simulink model "Balancing_Logic"  (R2023b)
settings: Solver=FixedStepDiscrete  StartTime=0.0  StopTime=Inf  RelTol=1e-3  EnableMultiTasking=on
values from neighbouring files (symbols this model uses):
  BalNotActWait = 30    [DD_Balancing_Logic.sldd]
  BalOffWait = 20    [DD_Balancing_Logic.sldd]
  BalOnWait = 60    [DD_Balancing_Logic.sldd]
  flgEnBalancing = 1    [DD_Balancing_Logic.sldd]
  TargetDeltaV = 0.01    [DD_Balancing_Logic.sldd]
undefined symbols (not defined in the file or in its folder): Ns
settings Model: DataDictionary=DD_Balancing_Logic.sldd  ExtModeTrigDuration=8  Creator=cpatel  LastModifiedBy=Alkhouly
settings SolverCC: AlgebraicLoopSolver=TrustRegion  AutoInsertRateTranBlk=on
settings DataIOCC: ExternalInput=Battery  SaveOutput=off  SaveTime=off  SignalLoggingName=logsOut
settings OptimizationCC: UseDivisionForNetSlopeComputation=on  UseFloatMulNetSlope=on  DefaultUnderspecifiedDataType=single  UseSpecifiedMinMax=on  PassReuseOutputArgsAs=Individual arguments  NoFixptDivByZeroProtection=on  EfficientFloat2IntCast=on  LifeSpan=inf  MaxStackSize=1024  OptimizeBlockOrder=speed  DifferentSizesBufferReuse=on  EfficientTunableParamExpr=on
settings DebuggingCC: SignalInfNanChecking=error  SaveWithParameterizedLinksMsg=none  CheckExecutionContextPreStartOutputMsg=on  IntegerOverflowMsg=error  ParameterPrecisionLossMsg=none  ParameterTunabilityLossMsg=error  UnconnectedInputMsg=warning  UnconnectedOutputMsg=warning  UnconnectedLineMsg=warning  AssertControl=DisableAll  PregeneratedLibrarySubsystemCodeDiagnostic=none  SFUnexpectedBacktrackingDiag=warning  SFNoUnconditionalDefaultTransitionDiag=warning  SFExecutionAtInitializationDiag=none  ArithmeticOperatorsInVariantConditions=warning
settings HardwareCC: ProdBitPerChar=16  ProdBitPerInt=16  ProdBitPerPointer=32  ProdBitPerSizeT=32  ProdBitPerPtrDiffT=32  ProdLargestAtomicInteger=Integer  ProdLargestAtomicFloat=None  ProdWordSize=16  ProdLongLongMode=on  ProdHWDeviceType=Texas Instruments->C2000  HardwareBoardFeatureSet=SoCBlockset
settings ModelReferenceCC: EnableRefExpFcnMdlSchedulingChecks=on  ModelReferenceNumInstancesAllowed=Single  PropagateSignalLabelsOutOfModel=off
settings SFSimCC: SimUseLocalCustomCode=off  MATLABDynamicMemAlloc=off  CustomCodeUndefinedFunction=UseInterfaceOnly
settings RTWCC: Description=Embedded Coder  SystemTargetFile=ert.tlc  HardwareBoard=TI Piccolo F280049C LaunchPad  GenCodeOnly=on  TemplateMakefile=ert_default_tmf  GenerateReport=on  RTWUseLocalCustomCode=off  Toolchain=Texas Instruments Code Composer Studio (C2000)  IncludeHyperlinkInReport=on  CodeProfilingSaveOptions=MetricsOnly  GenerateTraceInfo=on  GenerateTraceReport=on  GenerateTraceReportSl=on  GenerateTraceReportSf=on  GenerateTraceReportEml=on  GenerateWebview=on  GenerateCodeMetricsReport=on
settings CodeAppCC: ForceParamTrailComments=on  IgnoreCustomStorageClasses=off  MaxIdLength=51  OperatorAnnotations=on  SimulinkDataObjDesc=on  SFDataObjDesc=on  MangleLength=4  InsertBlockDesc=on  ReqsInCode=on
settings ERTTargetCC: CodeReplacementLibrary=TI C28x  UtilityFuncGeneration=Shared location  IncludeMdlTerminateFcn=off  CombineSignalStateStructs=on  SuppressErrorStatus=on  SupportNonFinite=off  SupportComplex=off  ParenthesesLevel=Maximum  CastingMode=Standards  GenerateSharedConstants=off  ExtModeTransport=4  ExtModeStaticAlloc=on  ExtModeAutomaticAllocSize=off  ExtModeStaticAllocSize=5000  ExtModeMexFile=ext_xcp  ExtModeIntrfLevel=Level2 - Open  PreserveExpressionOrder=on  PreserveIfCondition=on  EnableSignedLeftShifts=off  EnableSignedRightShifts=off
settings ConfigComp: CovMetricSettings=dcw  CovSaveCumulativeToWorkspaceVar=on  CovSaveSingleToWorkspaceVar=on  CovExternalEMLEnable=off  CovSFcnEnable=off  DVMode=DesignErrorDetection  DVMaxProcessTime=7000  DVTestSuiteOptimization=Auto  DVDetectDeadLogic=on  DVDetectIntegerOverflow=off

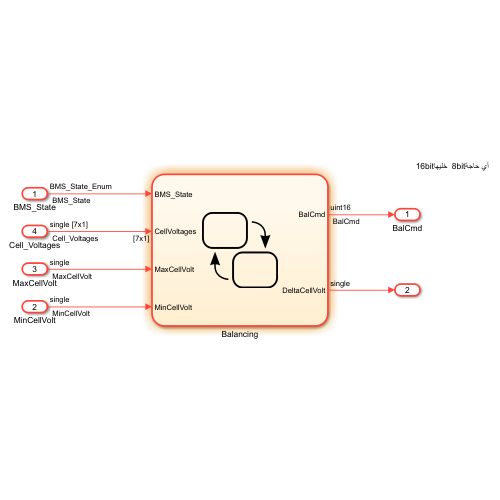
[thumbnail: Simulink's stored preview of the top-level diagram]
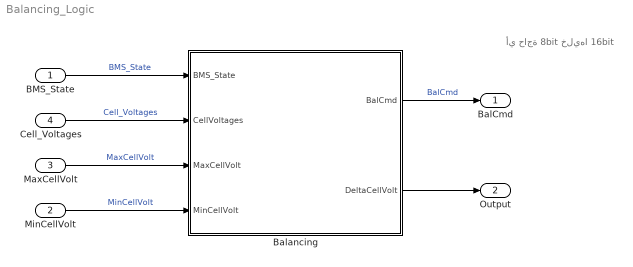
== system Balancing_Logic ==
  note: أي حاجة 8bit خليها 16bit
  BMS_State : Inport  OutDataTypeStr=Enum: BMS_State_Enum  PortDimensions=1  SampleTime=[5,0]
  MinCellVolt : Inport  Port=2  OutDataTypeStr=single  PortDimensions=1  SampleTime=[5,0]
  MaxCellVolt : Inport  Port=3  OutDataTypeStr=single  PortDimensions=1  SampleTime=[5,0]
  Cell_Voltages : Inport  Port=4  OutDataTypeStr=single  PortDimensions=[Ns 1]  SampleTime=[5,0]
  Balancing : Stateflow chart  TreatAsAtomicUnit=on  VariantControl=(default)
  BalCmd : Outport
  Output : Outport  Port=2
  wires:
  Balancing/1(BalCmd) -> BalCmd/1  "BalCmd"
  BMS_State/1 -> Balancing/1(BMS_State)  "BMS_State"
  MinCellVolt/1 -> Balancing/4(MinCellVolt)  "MinCellVolt"
  MaxCellVolt/1 -> Balancing/3(MaxCellVolt)  "MaxCellVolt"
  Cell_Voltages/1 -> Balancing/2(CellVoltages)  "Cell_Voltages"
  Balancing/2(DeltaCellVolt) -> Output/1

== stateflow chart Balancing_Logic/Balancing ==
  settings: updateMethod=DISCRETE  sampleTime=5
  state Balance [function]
    (default) -> (junction 504) : % Balance Command Update
    (junction 504) -> (junction 506) : {i=0;BalCmd=0;}
    (junction 506) -> (junction 505) [order 1] : [i<7]
    (junction 508) -> (junction 506)
    (junction 506) -> (junction 509) [order 2]
    (junction 505) -> (junction 507) : {BalCmd=BalCmd|(((CellVoltages[i] -MinCellVolt) >TargetDeltaV/2)<<i);}
    (junction 507) -> (junction 508) : {i=i+1;}
  state BalancingOFF
    en:
    BalCmd = 0;
    en,du:
    DeltaCellVolt = MaxCellVolt - MinCellVolt;
  state BalancingON
    en, du:
    DeltaCellVolt = MaxCellVolt - MinCellVolt;
    state BalActive
      en, du:
      Balance()
      flgBalCompl = (BalCmd>0);
    state BalNotActive
    (default) -> BalActive
    BalNotActive -> BalActive [order 1] : [after(BalNotActWait,sec) && ...
        | DeltaCellVolt > TargetDeltaV]
    BalActive -> BalNotActive : [flgBalCompl]
  (default) -> BalancingOFF : {flgBalCompl = true;}
  BalancingOFF -> BalancingON : [flgEnBalancing && ...
      | BMS_State ~= BMS_State_Enum.BMS_Driving && ...
      | after(BalOffWait,sec) && ...
      | DeltaCellVolt > TargetDeltaV]
  BalancingON -> BalancingOFF : [BMS_State == BMS_State_Enum.BMS_Driving] %In Driving State
  BalNotActive -> BalancingOFF [order 2] : [after(BalOnWait,sec)]
  data: BMS_State input Enum: BMS_State_Enum; CellVoltages input single; TargetDeltaV parameter; BalCmd output uint16 size=1 =uint16(0); flgBalCompl local uint16 size=1 =false; MaxCellVolt input single; MinCellVolt input single; BalNotActWait parameter; BalOffWait parameter; BalOnWait parameter; flgEnBalancing parameter; DeltaCellVolt output single size=1 =single(0); i local uint64
